simulink model "Milestone3_Battery"  (R2025b)
settings: Solver=VariableStepAuto  StartTime=0.0  StopTime=120  RelTol=1e-3
values from neighbouring files (symbols this model uses):
  C1 = 2000    [battery_params.m]    (also in simulinkmodel.m)
  OCV_vec = [3.0 3.25 3.35 3.4 3.45 3.6 3.7 3.85 3.95 4.05 4.15]    [battery_params.m]    (also in simulinkmodel.m = [3.00 3.40 3.60 3.80 4.20])
  Q_nom = 100    [battery_params.m]    (also in simulinkmodel.m = 5)
  R0 = 0.01    [battery_params.m]    (also in simulinkmodel.m = 0.05)
  R1 = 0.02    [battery_params.m]    (also in simulinkmodel.m = 0.01)
  SOC_init = 0.8    [battery_params.m]    (also in simulinkmodel.m = 0.9)
  SOC_max = 0.95    [battery_params.m]    (also in simulinkmodel.m = 1)
  SOC_min = 0.1    [battery_params.m]    (also in simulinkmodel.m = 0)
  SOC_vec = 0:0.1:1    [battery_params.m]    (also in simulinkmodel.m = [0 0.2 0.5 0.8 1])
settings Model: Creator=yousefmohamed

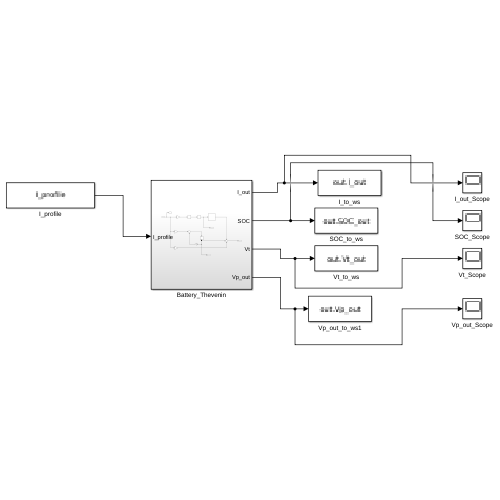
[thumbnail: Simulink's stored preview of the top-level diagram]
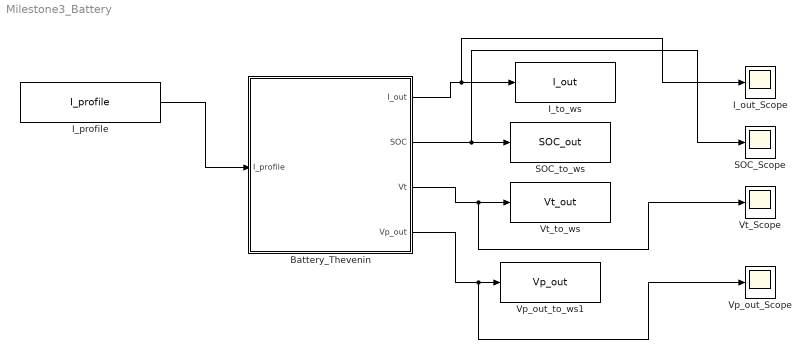
== system Milestone3_Battery ==
  Battery_Thevenin : Subsystem
  I_out_Scope : Scope
      settings: ActiveDisplayYMinimum=0.31250000000000006  ActiveDisplayYMaximum=2.1875
  I_profile : FromWorkspace  VariableName=I_profile
  I_to_ws : ToWorkspace  VariableName=I_out  SaveFormat=Structure With Time  SampleTime=-1
  SOC_Scope : Scope
      settings: ActiveDisplayYMinimum=0.89063454478107407  ActiveDisplayYMaximum=0.90104060613543624
  SOC_to_ws : ToWorkspace  VariableName=SOC_out  SaveFormat=Structure With Time  SampleTime=-1
  Vp_out_Scope : Scope
      settings: ActiveDisplayYMinimum=-0.0023977337300704624  ActiveDisplayYMaximum=0.021579603570634164  DataLoggingVariableName=ScopeData3
  Vp_out_to_ws1 : ToWorkspace  VariableName=Vp_out  SaveFormat=Structure With Time  SampleTime=-1
  Vt_Scope : Scope
      settings: ActiveDisplayYMinimum=3.8506944074917153  ActiveDisplayYMaximum=3.9888117325009205  DataLoggingVariableName=ScopeData2
  Vt_to_ws : ToWorkspace  VariableName=Vt_out  SaveFormat=Structure With Time  SampleTime=-1
  wires:
  I_profile/1 -> Battery_Thevenin/1(I_profile)
  Battery_Thevenin/3(Vt) -> Vt_Scope/1, Vt_to_ws/1
  Battery_Thevenin/2(SOC) -> SOC_Scope/1, SOC_to_ws/1
  Battery_Thevenin/1(I_out) -> I_out_Scope/1, I_to_ws/1
  Battery_Thevenin/4(Vp_out) -> Vp_out_Scope/1, Vp_out_to_ws1/1

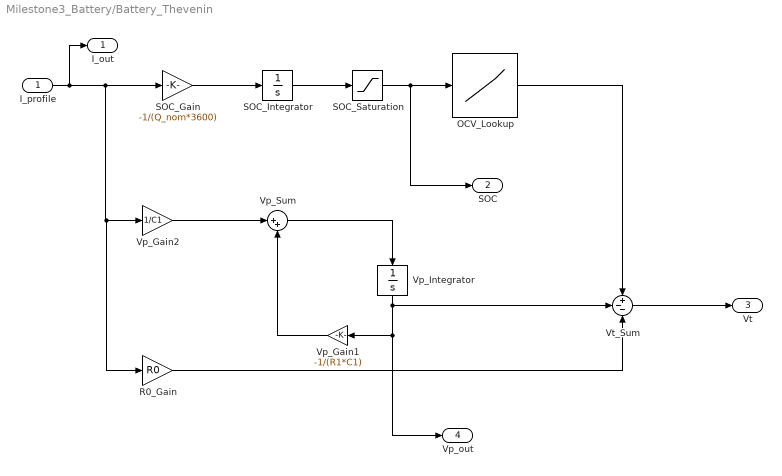
== system Milestone3_Battery/Battery_Thevenin ==
  I_profile : Inport
  OCV_Lookup : Lookup_n-D  NumberOfTableDimensions=1  BreakpointsForDimension1=SOC_vec  Table=OCV_vec  InternalRulePriority=Speed  RndMeth=Simplest
  R0_Gain : Gain  Gain=R0
  SOC_Gain : Gain  Gain=-1/(Q_nom*3600)
  SOC_Integrator : Integrator  InitialCondition=SOC_init
  SOC_Saturation : Saturate  UpperLimit=SOC_max  LowerLimit=SOC_min
  Vp_Gain1 : Gain  Gain=-1/(R1*C1)
  Vp_Gain2 : Gain  Gain=1/C1
  Vp_Integrator : Integrator
  Vp_Sum : Sum  Inputs=|++
  Vt_Sum : Sum  Inputs=+--
  I_out : Outport
  SOC : Outport  Port=2
  Vt : Outport  Port=3
  Vp_out : Outport  Port=4
  wires:
  I_profile/1 -> I_out/1, R0_Gain/1, Vp_Gain2/1, SOC_Gain/1
  SOC_Gain/1 -> SOC_Integrator/1
  SOC_Integrator/1 -> SOC_Saturation/1
  SOC_Saturation/1 -> SOC/1, OCV_Lookup/1
  Vp_Gain2/1 -> Vp_Sum/1
  Vp_Sum/1 -> Vp_Integrator/1
  Vp_Integrator/1 -> Vp_out/1, Vp_Gain1/1, Vt_Sum/2
  Vp_Gain1/1 -> Vp_Sum/2
  OCV_Lookup/1 -> Vt_Sum/1
  R0_Gain/1 -> Vt_Sum/3
  Vt_Sum/1 -> Vt/1
